simulink model "FilterCascade"  (R2020a)
settings: Solver=VariableStepAuto  StartTime=0.0  StopTime=10.0  RelTol=1e-3
libraries: simulink x1
settings Model: Creator=Hp  LastModifiedBy=Hp

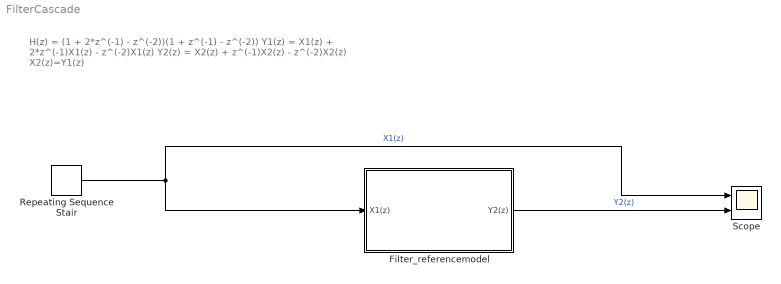
== system FilterCascade ==
  note: H(z) = (1 + 2*z^(-1) - z^(-2))(1 + z^(-1) - z^(-2))
      |
      | Y1(z) = X1(z) + 2*z^(-1)X1(z) - z^(-2)X1(z)
      | Y2(z) = X2(z) + z^(-1)X2(z) - z^(-2)X2(z)
      | X2(z)=Y1(z)
  Filter_referencemodel : Subsystem
  Repeating Sequence Stair : simulink/Sources/Repeating Sequence Stair  OutValues=[3 1 4 2 1].'  tsamp=0.1  OutMin=[]  OutMax=[]  OutDataTypeStr=double  OutputDataTypeScalingMode=double  OutDataType=fixdt(0,8)  ConRadixGroup=Best Precision: Vector-wise  OutScaling=2^-12
  Scope : Scope  NumInputPorts=2
  wires:
  Repeating Sequence Stair/1 -> Filter_referencemodel/1(X1(z)), Scope/1  "X1(z)"
  Filter_referencemodel/1(Y2(z)) -> Scope/2  "Y2(z)"

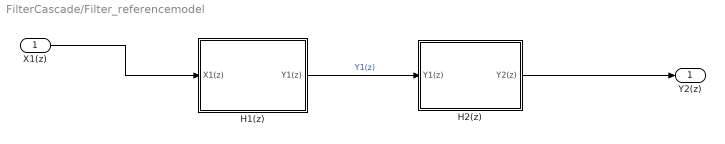
== system FilterCascade/Filter_referencemodel ==
  X1(z) : Inport
  H1(z) : Subsystem
  H2(z) : Subsystem
  Y2(z) : Outport
  wires:
  H1(z)/1(Y1(z)) -> H2(z)/1(Y1(z))  "Y1(z)"
  X1(z)/1 -> H1(z)/1(X1(z))
  H2(z)/1(Y2(z)) -> Y2(z)/1

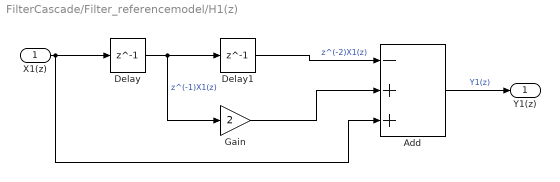
== system FilterCascade/Filter_referencemodel/H1(z) ==
  X1(z) : Inport
  Add : Sum  Inputs=-++
  Delay : Delay  DelayLength=1
  Delay1 : Delay  DelayLength=1
  Gain : Gain  Gain=2
  Y1(z) : Outport
  wires:
  Delay1/1 -> Add/1  "z^(-2)X1(z)"
  Delay/1 -> Gain/1, Delay1/1  "z^(-1)X1(z)"
  Add/1 -> Y1(z)/1  "Y1(z)"
  Gain/1 -> Add/2
  X1(z)/1 -> Add/3, Delay/1

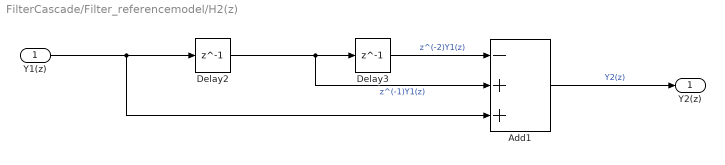
== system FilterCascade/Filter_referencemodel/H2(z) ==
  Y1(z) : Inport
  Add1 : Sum  Inputs=-++
  Delay2 : Delay  DelayLength=1
  Delay3 : Delay  DelayLength=1
  Y2(z) : Outport
  wires:
  Delay2/1 -> Add1/2, Delay3/1  "z^(-1)Y1(z)"
  Y1(z)/1 -> Add1/3, Delay2/1
  Delay3/1 -> Add1/1  "z^(-2)Y1(z)"
  Add1/1 -> Y2(z)/1  "Y2(z)"
